simulink model "is95revchtransmitter"  (Simulink 4.00)
settings: Solver=VariableStepDiscrete  SolverMode=SingleTasking  StartTime=0.0  StopTime=0.1  RelTol=1e-3  AbsTol=1e-6
undefined symbols (not defined in the file or in its folder): slcm
libraries: cdmalib x6, dspbdsp2 x3, dspsrcs2 x2, dspbuff2 x1
settings Model: Creator=rkumar  LastModifiedBy=agaltman  SaveTime=off  SaveOutput=off  LimitDataPoints=off  ExtModeTrigMode=oneshot  ExtModeArmWhenConnect=off  BlockReductionOpt=off

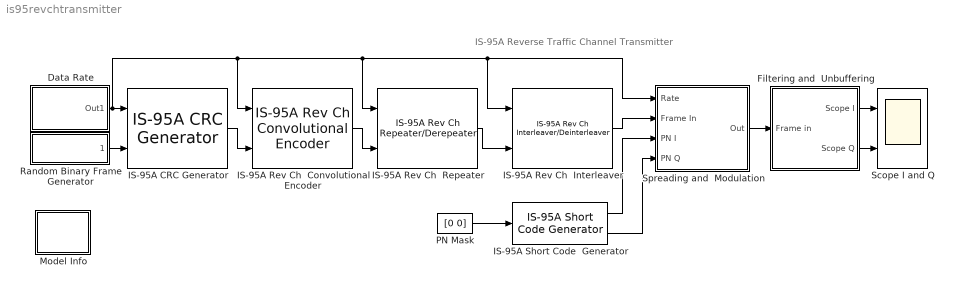
== system is95revchtransmitter ==
  note: IS-95A Reverse Traffic Channel Transmitter
  " Spreading and  Modulation" : Subsystem
      settings: RTWFcnNameOpts=Auto  RTWFileNameOpts=Auto
  Data Rate : Subsystem  mask{rate=Full}
      mask prompts: rate "Data Rate"
      settings: RTWFcnNameOpts=Auto  RTWFileNameOpts=Auto
      mask StyleString: popup(Full|Half|Quarter|One-Eighth)
      mask Display: disp('Mobile Station\n Transmitter \nData Rate')
  "Filtering and  Unbuffering " : Subsystem
      settings: RTWFcnNameOpts=Auto  RTWFileNameOpts=Auto
  IS-95A CRC Generator : cdmalib/IS-95A Common/IS-95A CRC Generator  rate_set=Rate Set I  ch_type=Traffic
  IS-95A Rev Ch  Convolutional Encoder : cdmalib/IS-95A Mobile Station Transmitter/IS-95A Rev Ch Convolutional Encoder  rate_set=Rate Set I  ch_type=Traffic  enc_state=[]
  IS-95A Rev Ch  Interleaver : cdmalib/IS-95A Mobile Station Transmitter/IS-95A Rev Ch Interleaver//Deinterleaver  ch_type=Traffic  int_select=Interleaver
  IS-95A Rev Ch  Repeater : cdmalib/IS-95A Mobile Station Transmitter/IS-95A Rev Ch Repeater//Derepeater  ch_type=Traffic  rep_select=Derepeater
  IS-95A Short Code  Generator : cdmalib/IS-95A Common/IS-95A Short Code Generator  numOut=64  sampTime=1/(50*384)
  Model Info : Subsystem  LoadFcn=slcm LoadBlock;  InitFcn=slcm('UpdateAllCMBlocksInThisModelInit')  mask(CMBlock){InitialSaveTempField=, InitialBlockCM=none, BlockCM=none, Frame=on, SaveTempField=, DisplayStringWithTags=Info, MaskDisplayString=Info, HorizontalTextAlignment=Center, LeftAlignmentValue=0.5, SourceBlockDiagram=is95revchtransmitter, TagMaxNumber=20, CMTag1=, CMTag2=, CMTag3=, CMTag4=, CMTag5=, CMTag6=, CMTag7=, CMTag8=, CMTag9=, CMTag10=, CMTag11=, CMTag12=, CMTag13=, CMTag14=, CMTag15=, CMTag16=, CMTag17=, CMTag18=, CMTag19=, CMTag20=}
      mask help: This block allows revision control information to be displayed within the model.
      settings: CopyFcn=slcm CopyBlock;  DeleteFcn=slcm Cancel;  PostSaveFcn=slcm('UpdateAllCMBlocksInThisModel')  NameChangeFcn=slcm Rename;  OpenFcn=cdmademohelp;  RTWFcnNameOpts=Auto  RTWFileNameOpts=Auto
      mask Display: text(str2num(LeftAlignmentValue), 0.5, MaskDisplayString, 'HorizontalAlignment', HorizontalTextAlignment)
  PN Mask : Constant  Value=[0 0]
  Random Binary Frame Generator : Subsystem  mask(Random Binary Frame Generator){seed=119940, Ts=1/(50*268), N=268}
      mask prompts: seed "Initial seed:"; Ts "Sample time (sec):"; N "Ouput frame size:"
      settings: RTWFcnNameOpts=Auto  RTWFileNameOpts=Auto
      mask Display: plot(0,0,100,100,[95,90,90,80,80,60,60,30,30,20,20,10,10,5],[25,25,75,75,25,25,75,75,25,25,75,75,25,25]);
  Scope I and Q : Scope  NumInputPorts=2
      settings: TickLabels=on  TimeRange=0.0001  YMin=-2~-2  YMax=2~2  SaveToWorkspace=off  SaveName=ScopeData  DataFormat=Array  LimitDataPoints=on  MaxDataPoints=5000
  wires:
  IS-95A Rev Ch  Convolutional Encoder/1 -> IS-95A Rev Ch  Repeater/2
  IS-95A CRC Generator/1 -> IS-95A Rev Ch  Convolutional Encoder/2
  IS-95A Rev Ch  Repeater/1 -> IS-95A Rev Ch  Interleaver/2
  IS-95A Rev Ch  Interleaver/1 -> " Spreading and  Modulation"/2(Frame In)
  PN Mask/1 -> IS-95A Short Code  Generator/1
  IS-95A Short Code  Generator/1 -> " Spreading and  Modulation"/3(PN I)
  IS-95A Short Code  Generator/2 -> " Spreading and  Modulation"/4(PN Q)
  "Filtering and  Unbuffering "/1(Scope I) -> Scope I and Q/1
  "Filtering and  Unbuffering "/2(Scope Q) -> Scope I and Q/2
  Random Binary Frame Generator/1(" ") -> IS-95A CRC Generator/2
  Data Rate/1(Out1) -> IS-95A Rev Ch  Convolutional Encoder/1, IS-95A Rev Ch  Repeater/1, IS-95A Rev Ch  Interleaver/1, " Spreading and  Modulation"/1(Rate), IS-95A CRC Generator/1
  " Spreading and  Modulation"/1("Out ") -> "Filtering and  Unbuffering "/1(Frame in)

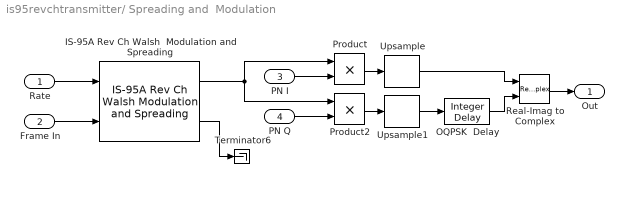
== system is95revchtransmitter/ Spreading and  Modulation ==
  Rate : Inport  Port=1
  Frame In : Inport  Port=2
  PN I : Inport  Port=3
  PN Q : Inport  Port=4
  IS-95A Rev Ch Walsh  Modulation and Spreading : cdmalib/IS-95A Mobile Station Transmitter/IS-95A Rev Ch Walsh Modulation and Spreading  chType=Traffic  lngCdMask=1  wlshOrd=6  sampTime=1/(50*384)
  OQPSK  Delay : dspbdsp2/Integer Delay  delay=4  ic=0  frame=on  df=on  numChans=1
  Product : Product  Inputs=2  Multiplication=Element-wise(.*)  SaturateOnIntegerOverflow=on
  Product2 : Product  Inputs=2  Multiplication=Element-wise(.*)  SaturateOnIntegerOverflow=on
  Real-Imag to Complex : RealImagToComplex  Input=RealAndImag  ConstantPart=0
  Terminator6 : Terminator
  Upsample : dspbdsp2/Upsample  N=8  phase=0  ic=0  frame=on  nchans=1  mode=Maintain input frame rate
  Upsample1 : dspbdsp2/Upsample  N=8  phase=0  ic=0  frame=on  nchans=1  mode=Maintain input frame rate
  "Out " : Outport  Port=1
  wires:
  Real-Imag to Complex/1 -> "Out "/1
  Upsample/1 -> Real-Imag to Complex/1
  OQPSK  Delay/1 -> Real-Imag to Complex/2
  Upsample1/1 -> OQPSK  Delay/1
  Product2/1 -> Upsample1/1
  Product/1 -> Upsample/1
  PN Q/1 -> Product2/2
  Frame In/1 -> IS-95A Rev Ch Walsh  Modulation and Spreading/2
  IS-95A Rev Ch Walsh  Modulation and Spreading/2 -> Terminator6/1
  PN I/1 -> Product/2
  Rate/1 -> IS-95A Rev Ch Walsh  Modulation and Spreading/1
  IS-95A Rev Ch Walsh  Modulation and Spreading/1 -> Product2/1, Product/1

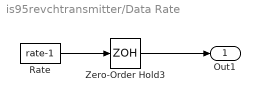
== system is95revchtransmitter/Data Rate ==
  Rate : Constant  Value=rate-1
  Zero-Order Hold3 : ZeroOrderHold  SampleTime=1/50
  Out1 : Outport  Port=1  InitialOutput=0
  wires:
  Zero-Order Hold3/1 -> Out1/1
  Rate/1 -> Zero-Order Hold3/1

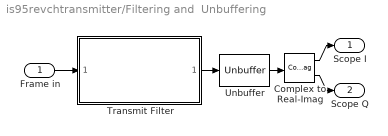
== system is95revchtransmitter/Filtering and  Unbuffering  ==
  Frame in : Inport  Port=1
  Complex to Real-Imag : ComplexToRealImag  Output=RealAndImag
  Transmit Filter : Subsystem  mask(FIR Pulse Shaping Filter){N=1}
      mask prompts: N "Interpolation factor:"
      mask help: The length of the FIR filter is the duration of 12 PN sequence chips. The coefficient spacing and the sample time of this filter is one-eighth of the PN sequence chip duration, resulting in a total of 96 coefficients. The filter introduces a delay of 48 samples.
      mask init:
      | load txfiltx8.mat;
      | h = (TxFiltCoefx8*N);
      settings: RTWFcnNameOpts=Auto  RTWFileNameOpts=Auto
      mask Display: plot( 1:prod( size( h)), h);
  Unbuffer : dspbuff2/Unbuffer  ic=0  num_chans=1
  Scope I : Outport  Port=1
  Scope Q : Outport  Port=2
  wires:
  Frame in/1 -> Transmit Filter/1("   ")
  Transmit Filter/1(" ") -> Unbuffer/1
  Unbuffer/1 -> Complex to Real-Imag/1
  Complex to Real-Imag/1 -> Scope I/1
  Complex to Real-Imag/2 -> Scope Q/1

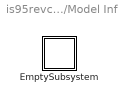
== system is95revchtransmitter/Model Info ==
  EmptySubsystem : Subsystem
      settings: RTWFcnNameOpts=Auto  RTWFileNameOpts=Auto

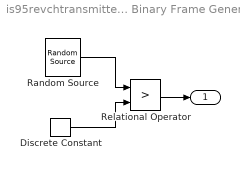
== system is95revchtransmitter/Random Binary Frame Generator ==
  Discrete Constant : dspsrcs2/Discrete Constant  Value=0.5  Ts=Ts*N
  Random Source : dspsrcs2/Random Source  SrcType=Uniform  Min=0  Max=1  Mean=0  Var=1  Seed=seed  SampMode=Discrete  Inherit=off  SampTime=Ts  SampFrame=N  OutComplex=Real
  Relational Operator : RelationalOperator  Operator=>
  " " : Outport  Port=1
  wires:
  Random Source/1 -> Relational Operator/1
  Discrete Constant/1 -> Relational Operator/2
  Relational Operator/1 -> " "/1

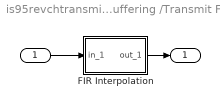
== system is95revchtransmitter/Filtering and  Unbuffering /Transmit Filter ==
  "   " : Inport  Port=1
  FIR Interpolation : Subsystem  mask(FIR Interpolation){h=h, L=N, frame=on, numChans=1, framing=Maintain input frame rate}
      mask prompts: h "FIR filter coefficients:"; L "Interpolation factor:"; frame "Frame-based inputs"; numChans "Number of channels:"
      mask help: Upsample input signal by an integer factor, then apply an FIR filter. Implemented using an efficient polyphase interpolation structure. The filter coefficients are scaled by the interpolation factor.
      mask init:
      | outputBufInitCond = 0;
      | [str,numChans] = dspblkupfir('setup1',numChans);
      | [h,framing,str]= dspblkupfir('setup2',h,L,framing);
      settings: RTWFcnNameOpts=Auto  RTWFileNameOpts=Auto
      mask Help: web(dspbhelp);
      mask StyleString: edit,edit,checkbox,edit,popup(Maintain input frame size|Maintain input frame rate)
      mask CallbackString: ||dspblkupfir||
      mask Display: disp(str)
  " " : Outport  Port=1
  wires:
  "   "/1 -> FIR Interpolation/1(in_1)
  FIR Interpolation/1(out_1) -> " "/1

== system is95revchtransmitter/Model Info/EmptySubsystem ==

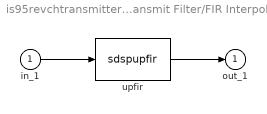
== system is95revchtransmitter/Filtering and  Unbuffering /Transmit Filter/FIR Interpolation ==
  in_1 : Inport  Port=1
  upfir : S-Function  FunctionName=sdspupfir  Parameters=h,L,numChans,framing,outputBufInitCond  PortCounts=[]  SFunctionModules=''
  out_1 : Outport  Port=1  InitialOutput=0
  wires:
  upfir/1 -> out_1/1
  in_1/1 -> upfir/1
